simulink model "rtwdemo_codetemplate"  (Simulink 6.0)
settings: Solver=FixedStepDiscrete  StartTime=0.0  StopTime=48  FixedStep=1  RelTol=1e-3
libraries: rtwdemowidgets x2
settings Model: CovMetricSettings=d  Creator=The MathWorks Inc.  LastModifiedBy=batserve  ParamWorkspaceSource=ReferencedWorkspace  ExtModeTrigMode=oneshot  ExtModeArmWhenConnect=off  ExtModeAutoUpdateStatusClock=off
settings DataIOCC: LimitDataPoints=off  SaveFormat=StructureWithTime  SaveOutput=off  SaveTime=off  SignalLoggingName=sigsOut
settings OptimizationCC: InlineParams=on  EnforceIntegerDowncast=off  StateBitsets=on  DataBitsets=on  UseTempVars=on  ZeroExternalMemoryAtStartup=off  ZeroInternalMemoryAtStartup=off  InitFltsAndDblsToZero=off  NoFixptDivByZeroProtection=on  OptimizeModelRefInitCode=on  LifeSpan=1
settings DebuggingCC: CheckExecutionContextPreStartOutputMsg=on  CheckExecutionContextRuntimeOutputMsg=on  SolverPrmCheckMsg=none  IntegerOverflowMsg=none
settings ModelReferenceCC: UpdateModelReferenceTargets=IfOutOfDate
settings RTWCC: SystemTargetFile=ert.tlc  TLCOptions=-p0 -aWarnNonSaturatedBlocks=0  TemplateMakefile=ert_default_tmf  GenerateReport=on  RTWVerbose=off  ProcessScript=ert_make_rtw_hook  IncludeHyperlinkInReport=on  LaunchReport=on
settings CodeAppCC: ForceParamTrailComments=on  IgnoreCustomStorageClasses=off  SimulinkDataObjDesc=on  PrefixModelToSubsysFcnNames=off  CustomSymbolStr=$N$M  InsertBlockDesc=on
settings ERTTargetCC: TargetFcnLib=ansi_tfl_tmw.mat  GenFloatMathFcnCalls=ANSI_C  GenerateSampleERTMain=on  IncludeMdlTerminateFcn=off  SupportNonFinite=off  SupportComplex=off  InlinedParameterPlacement=NonHierarchical  RootIOFormat=Individual Arguments  ERTSrcFileBannerTemplate=rtwdemocodetemplate.cgt  ERTHdrFileBannerTemplate=rtwdemocodetemplate.cgt  ERTDataSrcFileTemplate=rtwdemocodetemplate.cgt  ERTDataHdrFileTemplate=rtwdemocodetemplate.cgt  ERTCustomFileTemplate=example_file_process.tlc  InitialValueSource=Model

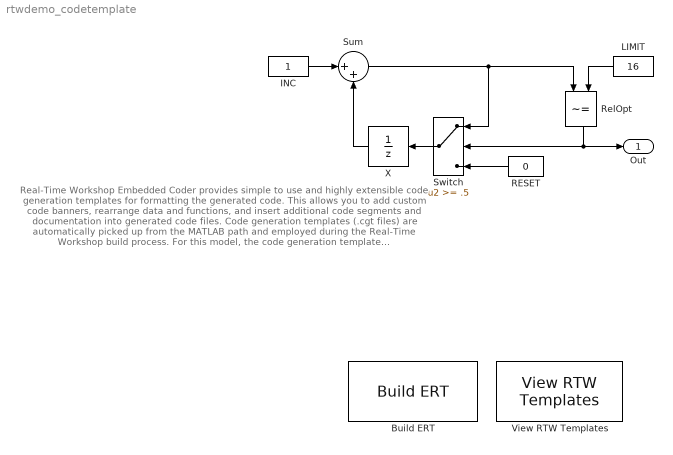
== system rtwdemo_codetemplate ==
  note: Real-Time Workshop Embedded Coder provides simple to use and highly extensible code
      | generation templates for formatting the generated code.  This allows you to add custom
      | code banners, rearrange data and functions, and insert additional code segments and
      | documentation into generated code files.  Code generation templates (.cgt files) are
      | automatically picked up from the MATLAB path and employed during the Real-Time Workshop
      | build process.  For this model, the code generation template rtwdemocodetemplate.cgt
      | is specified in the Configuration Parameters->Templates page.  Launch the templates
      | page from the yellow button below and press edit for the listed templates.
  Build ERT : rtwdemowidgets/Build ERT  attrib_overrides={'ERTSrcFileBannerTemplate', 'ERTHdrFileBannerTemplate', 'ERTDataSrcFileTemplate', 'ERTDataHdrFileTemplate'}
  INC : Constant  OutDataTypeMode=uint8
  LIMIT : Constant  Orientation=left  Value=16  OutDataTypeMode=uint8
  RESET : Constant  Orientation=left  Value=0  OutDataTypeMode=uint8
  RelOpt : RelationalOperator  Orientation=down  Operator=~=  InputSameDT=on
  Sum : Sum  Inputs=|++  InputSameDT=on
  Switch : Switch  Orientation=left  Threshold=.5  SaturateOnIntegerOverflow=on  InputSameDT=on
  View RTW Templates : rtwdemowidgets/View RTW Templates
  X : UnitDelay  Orientation=left  StateIdentifier=X
  Out : Outport
  wires:
  INC/1 -> Sum/1
  X/1 -> Sum/2
  Switch/1 -> X/1
  Sum/1 -> Switch/1, RelOpt/1
  LIMIT/1 -> RelOpt/2
  RESET/1 -> Switch/3
  RelOpt/1 -> Switch/2, Out/1
